simulink model "ARO40506DOF_2020a_2025"  (R2025b)
settings: Solver=FixedStepAuto  StartTime=0.0  StopTime=60  FixedStep=.01  RelTol=1e-3
libraries: simulink_extras x7
settings Model: PacingRate=1000  Creator=Rainman  LastModifiedBy=cdriggs
settings SolverCC: ZeroCrossControl=EnableAll
settings DebuggingCC: SignalInfNanChecking=warning
settings RTWCC: GPUComputeCapability=3.5

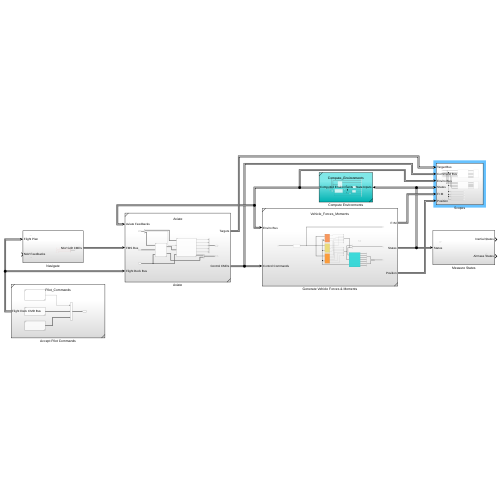
[thumbnail: Simulink's stored preview of the top-level diagram]
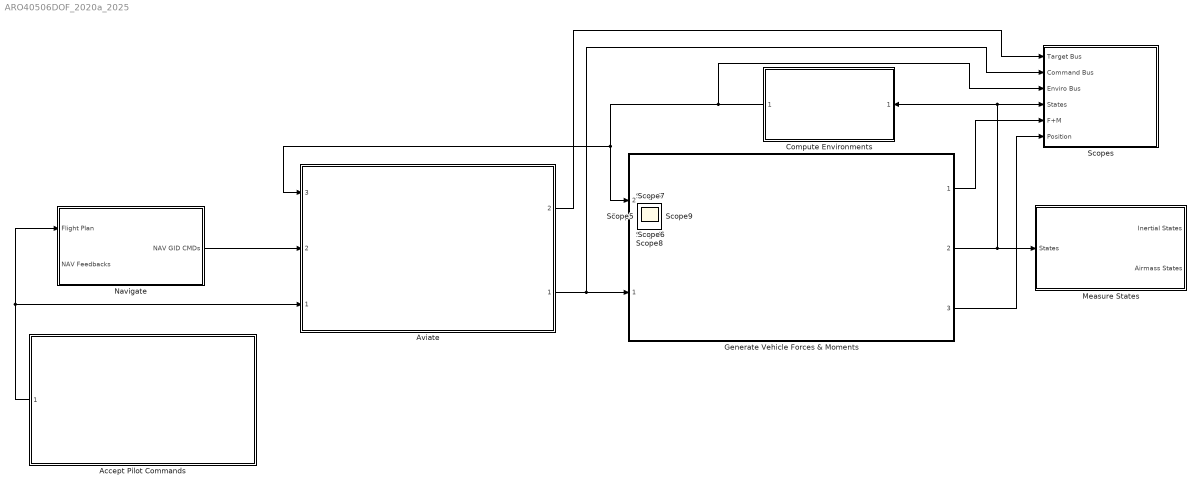
== system ARO40506DOF_2020a_2025 ==
  Accept Pilot Commands : Subsystem  ReferencedSubsystem=Pilot_Commands
  Aviate : Subsystem  ReferencedSubsystem=Aviate
      settings: PortSchema="{\"entries\":[{\"content\":{\"sides\":[{\"content\":{\"connectorIds\":[\"In3\",\"In2\",\"In1\"]},\"type\":\"ConnectorPlacement.EquallySpacedRectSide\",\"uuid\":\"f13bb7a0-c278-4e6a-87bd-80b067821608\"},{\"content\":{\"connectorIds\":[\"Out2\",\"Out1\"],\"side\":\"RIGHT\"},\"type\":\"ConnectorPlacement.EquallySpacedRectSide\",\"uuid\":\"000ddb2c-cb93-4942-87ef-30ae2dcc275e\"},{\"content\":{\"side\":\"TOP\"},\"type\":\"ConnectorPlacement.EquallySpacedRectSide\",\"uuid\":\"c3152a53-2ce1-4a0b-9ad8-bcbeca850b30\"}]},\"type\":\"ConnectorPlacement.EquallySpacedConnector\",\"uuid\":\"e0cd03c4-ca4d-4b0c-94c1-0c67997df9b9\"}],\"packageUris\":[\"http://schema.mathworks.com/mf0/Connector/R2020b\"],\"version\":\"1.0\"}"
  Compute Environments : Subsystem  ReferencedSubsystem=Compute_Environments
  Generate Vehicle Forces & Moments : Subsystem  ReferencedSubsystem=Vehicle_Forces_Moments
      settings: PortSchema="{\"entries\":[{\"content\":{\"sides\":[{\"content\":{\"connectorIds\":[\"In2\",\"In1\"]},\"type\":\"ConnectorPlacement.EquallySpacedRectSide\",\"uuid\":\"c7a215e5-d416-4ad4-83d0-8365272d1a03\"},{\"content\":{\"connectorIds\":[\"Out1\",\"Out2\",\"Out3\"],\"side\":\"RIGHT\"},\"type\":\"ConnectorPlacement.EquallySpacedRectSide\",\"uuid\":\"c94239bd-91e1-4e40-88df-9a8012874706\"},{\"content\":{\"side\":\"TOP\"},\"type\":\"ConnectorPlacement.EquallySpacedRectSide\",\"uuid\":\"517c4bf5-dd91-4ac4-b774-658dcc3846ed\"}]},\"type\":\"ConnectorPlacement.EquallySpacedConnector\",\"uuid\":\"ee7d0a5a-600e-4f04-ae5a-149fcc3f5966\"}],\"packageUris\":[\"http://schema.mathworks.com/mf0/Connector/R2020b\"],\"version\":\"1.0\"}"
  Measure States : Subsystem
  Navigate : Subsystem
  Scopes : Subsystem
  Scope{,1..9} (10 alike) : Scope
      Scope settings: ActiveDisplayYMinimum=824.79015242294952  ActiveDisplayYMaximum=887.11668658276335  DataLoggingVariableName=ScopeData16
      Scope1 settings: ActiveDisplayYMinimum=-0.0918699619645163  ActiveDisplayYMaximum=0.1361905923482078  DataLoggingVariableName=ScopeData17
      Scope2 settings: ActiveDisplayYMinimum=-0.0012525958255160388  ActiveDisplayYMaximum=0.0018610833356130711  DataLoggingVariableName=ScopeData18
      Scope3 settings: ActiveDisplayYMinimum=-1  ActiveDisplayYMaximum=1  DataLoggingVariableName=ScopeData8
      Scope4 settings: ActiveDisplayYMinimum=-1  ActiveDisplayYMaximum=1  DataLoggingVariableName=ScopeData19
      Scope5 settings: ActiveDisplayYMinimum=-1  ActiveDisplayYMaximum=1  DataLoggingVariableName=ScopeData8
      Scope6 settings: ActiveDisplayYMinimum=-1  ActiveDisplayYMaximum=1  DataLoggingVariableName=ScopeData19
      Scope7 settings: ActiveDisplayYMinimum=-10.79844220865172  ActiveDisplayYMaximum=12.310938023183525  DataLoggingVariableName=ScopeData24
      Scope8 settings: ActiveDisplayYMinimum=-2.0057474745908946E-6  ActiveDisplayYMaximum=1.8051727271318056E-5  DataLoggingVariableName=ScopeData25
      Scope9 settings: ActiveDisplayYMinimum=-1.1579459752656034  ActiveDisplayYMaximum=0.3943110608301495  DataLoggingVariableName=ScopeData29
  wires:
  Navigate/1(NAV GID CMDs) -> Aviate/2
  Aviate/1 -> Scopes/2(Command Bus), Generate Vehicle Forces & Moments/1
  Accept Pilot Commands/1 -> Navigate/1(Flight Plan), Aviate/1
  Generate Vehicle Forces & Moments/2 -> Compute Environments/1, Scopes/4(States), Measure States/1(States)
  Compute Environments/1 -> Scopes/3(Enviro Bus), Generate Vehicle Forces & Moments/2, Aviate/3
  Generate Vehicle Forces & Moments/1 -> Scopes/5(F+M)
  Generate Vehicle Forces & Moments/3 -> Scopes/6(Position)
  Aviate/2 -> Scopes/1(Target Bus)

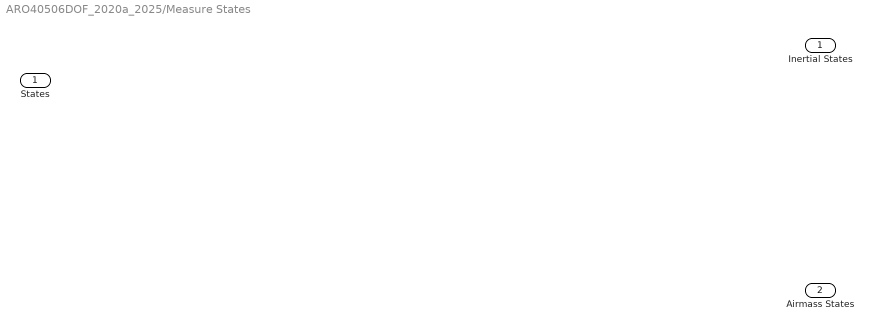
== system ARO40506DOF_2020a_2025/Measure States ==
  States : Inport
  Inertial States : Outport
  Airmass States : Outport  Port=2

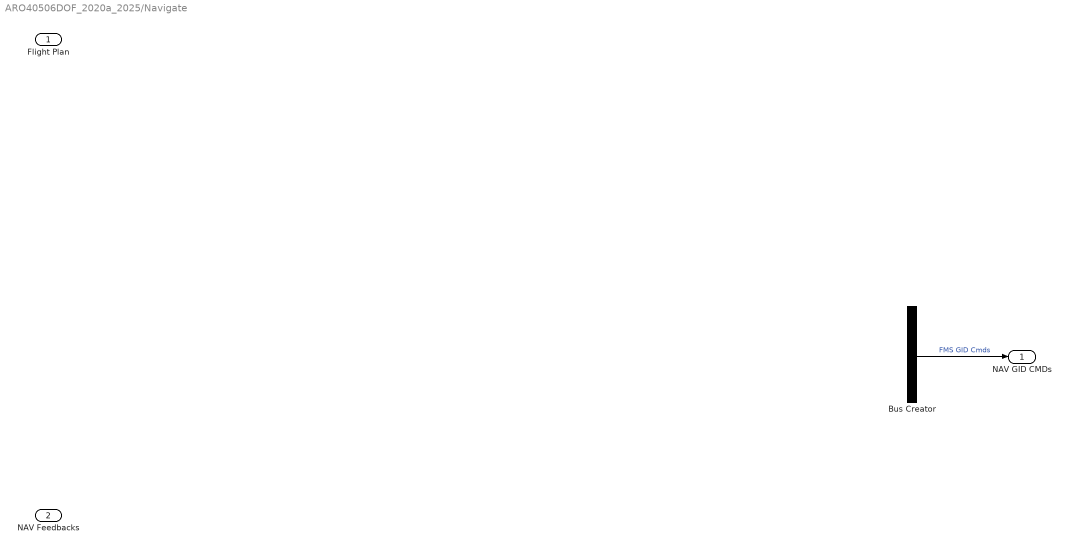
== system ARO40506DOF_2020a_2025/Navigate ==
  Flight Plan : Inport
  NAV Feedbacks : Inport  Port=2
  Bus Creator : BusCreator  Inputs=4
  NAV GID CMDs : Outport
  wires:
  Bus Creator/1 -> NAV GID CMDs/1  "FMS GID Cmds"
  ? -> Bus Creator/1  "FMS ALT Target"
  ? -> Bus Creator/2  "FMS VS Target"
  ? -> Bus Creator/3  "FMS HDG Target"
  ? -> Bus Creator/4  "FMS SPD Target"

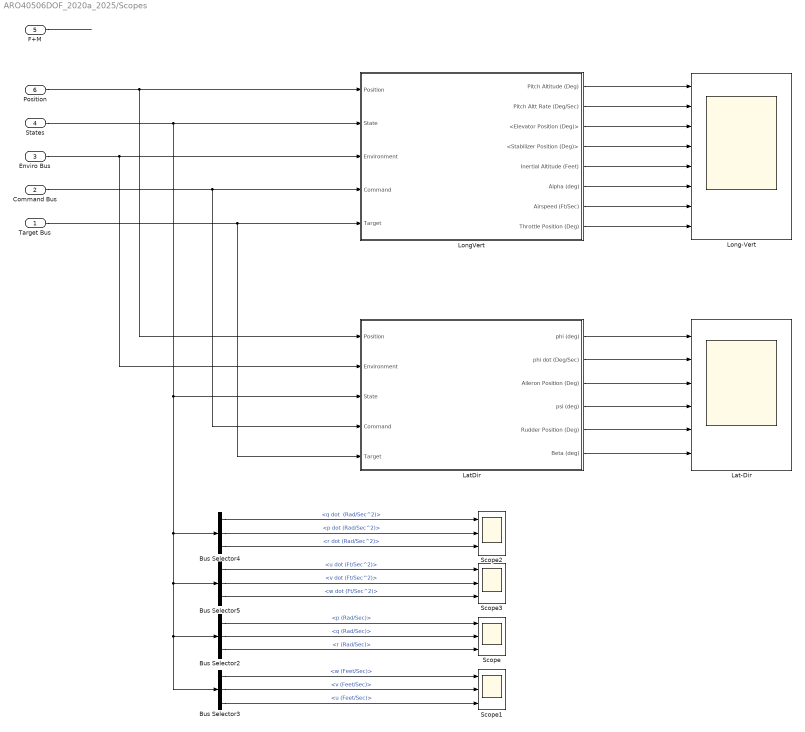
== system ARO40506DOF_2020a_2025/Scopes ==
  Target Bus : Inport
  Command Bus : Inport  Port=2
  Enviro Bus : Inport  Port=3
  States : Inport  Port=4
  F+M : Inport  Port=5
  Position : Inport  Port=6
  Bus Selector2 : BusSelector  OutputSignals=Rotat.Body.Rates (Rad/Sec).p (Rad/Sec),Rotat.Body.Rates (Rad/Sec).q (Rad/Sec),Rotat.Body.Rates (Rad/Sec).r (Rad/Sec)
  Bus Selector3 : BusSelector  OutputSignals=Trans.Body Veloc.w (Feet/Sec),Trans.Body Veloc.v (Feet/Sec),Trans.Body Veloc.u (Feet/Sec)
  Bus Selector4 : BusSelector  OutputSignals="Rotat.Body.Accelerations (Rad/Sec^2).q dot  (Rad/Sec^2),Rotat.Body.Accelerations (Rad/Sec^2).p dot (Rad/Sec^2),Rotat.Body.Accelerations (Rad/Sec^2).r dot (Rad/Sec^2)"
  Bus Selector5 : BusSelector  OutputSignals=Trans.Lin Accels.u dot (Ft/Sec^2),Trans.Lin Accels.v dot (Ft/Sec^2),Trans.Lin Accels.w dot (Ft/Sec^2)
  Lat-Dir : Scope  NumInputPorts=6
      settings: ActiveDisplayYMinimum=-6.499523495214234  ActiveDisplayYMaximum=17.811539807152641
  LatDir : Subsystem
  Long-Vert : Scope  NumInputPorts=8
      settings: ActiveDisplayYMinimum=-0.011330669657011287  ActiveDisplayYMaximum=0.010438336756237168
  LongVert : Subsystem
  Scope{,1..3} (4 alike) : Scope  NumInputPorts=3
      Scope settings: ActiveDisplayYMinimum=-5.25071638692835E-14  ActiveDisplayYMaximum=8.1502400193216538E-14  DataLoggingVariableName=ScopeData2
      Scope1 settings: ActiveDisplayYMinimum=-80.784705727324493  ActiveDisplayYMaximum=49.537985206955256  DataLoggingVariableName=ScopeData3
      Scope2 settings: ActiveDisplayYMinimum=-0.010938926120745193  ActiveDisplayYMaximum=0.089546281056735608  DataLoggingVariableName=ScopeData6
      Scope3 settings: ActiveDisplayYMinimum=-7.3926575931100222  ActiveDisplayYMaximum=3.2145324083165696  DataLoggingVariableName=ScopeData9
  wires:
  States/1 -> LongVert/2(State), LatDir/3(State), Bus Selector4/1, Bus Selector5/1, Bus Selector2/1, Bus Selector3/1
  Enviro Bus/1 -> LatDir/2(Environment), LongVert/3(Environment)
  Bus Selector2/1 -> Scope/1  "<p (Rad/Sec)>"
  Bus Selector2/2 -> Scope/2  "<q (Rad/Sec)>"
  Bus Selector2/3 -> Scope/3  "<r (Rad/Sec)>"
  Bus Selector3/1 -> Scope1/1  "<w (Feet/Sec)>"
  Bus Selector3/2 -> Scope1/2  "<v (Feet/Sec)>"
  Bus Selector3/3 -> Scope1/3  "<u (Feet/Sec)>"
  Bus Selector4/2 -> Scope2/2  "<p dot (Rad/Sec^2)>"
  Bus Selector4/3 -> Scope2/3  "<r dot (Rad/Sec^2)>"
  Bus Selector4/1 -> Scope2/1  "<q dot  (Rad/Sec^2)>"
  Bus Selector5/1 -> Scope3/1  "<u dot (Ft/Sec^2)>"
  Bus Selector5/2 -> Scope3/2  "<v dot (Ft/Sec^2)>"
  Bus Selector5/3 -> Scope3/3  "<w dot (Ft/Sec^2)>"
  F+M/1 -> ?
  Position/1 -> LatDir/1(Position), LongVert/1(Position)
  LongVert/1(Pitch Altitude (Deg)) -> Long-Vert/1
  LongVert/2(Pitch Altt Rate (Deg/Sec)) -> Long-Vert/2
  LongVert/3(<Elevator Position (Deg)>) -> Long-Vert/3
  LongVert/4(<Stabilizer Position (Deg)>) -> Long-Vert/4
  LongVert/5(Inertial Altitude (Feet)) -> Long-Vert/5
  LongVert/6(Alpha (deg)) -> Long-Vert/6
  LongVert/7(Airspeed (Ft/Sec)) -> Long-Vert/7
  LongVert/8(Throttle Position (Deg)) -> Long-Vert/8
  LatDir/1(phi (deg)) -> Lat-Dir/1
  LatDir/2(phi dot (Deg/Sec)) -> Lat-Dir/2
  LatDir/3(Aileron Position (Deg)) -> Lat-Dir/3
  LatDir/4(psi (deg)) -> Lat-Dir/4
  LatDir/5(Rudder Position (Deg)) -> Lat-Dir/5
  LatDir/6(Beta (deg)) -> Lat-Dir/6
  Command Bus/1 -> LongVert/4(Command), LatDir/4(Command)
  Target Bus/1 -> LatDir/5(Target), LongVert/5("Target ")

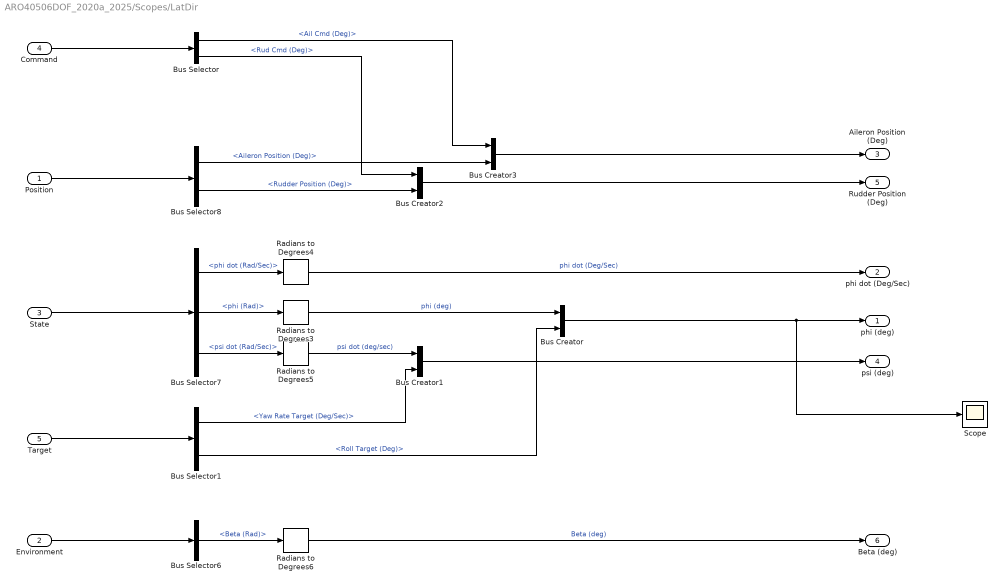
== system ARO40506DOF_2020a_2025/Scopes/LatDir ==
  Position : Inport
  Environment : Inport  Port=2
  State : Inport  Port=3
  Command : Inport  Port=4
  Target : Inport  Port=5
  Bus Creator{,1..3} (4 alike) : BusCreator  Inputs=2
  Bus Selector : BusSelector  OutputSignals=Ail Cmd (Deg),Rud Cmd (Deg)
  Bus Selector1 : BusSelector  OutputSignals=signal1.Yaw Rate Target (Deg/Sec),signal1.Roll Target (Deg)
  Bus Selector6 : BusSelector  OutputSignals=Aero angles.Beta (Rad)
  Bus Selector7 : BusSelector  OutputSignals=Rotat.Attitude Rates.phi dot (Rad/Sec),Rotat.Attitude.phi (Rad),Rotat.Attitude Rates.psi dot (Rad/Sec)
  Bus Selector8 : BusSelector  OutputSignals=Aileron Position (Deg),Rudder Position (Deg)
  Radians to Degrees{3..6} (4 alike) : simulink_extras/Transformations/Radians to Degrees
  Scope : Scope
      settings: ActiveDisplayYMinimum=-1  ActiveDisplayYMaximum=1  DataLoggingVariableName=ScopeData27
  phi (deg) : Outport
  phi dot (Deg/Sec) : Outport  Port=2
  Aileron Position (Deg) : Outport  Port=3
  psi (deg) : Outport  Port=4
  Rudder Position (Deg) : Outport  Port=5
  Beta (deg) : Outport  Port=6
  wires:
  Radians to Degrees3/1 -> Bus Creator/1  "phi (deg)"
  Bus Creator1/1 -> psi (deg)/1
  Bus Selector/1 -> Bus Creator3/1  "<Ail Cmd (Deg)>"
  Bus Selector6/1 -> Radians to Degrees6/1  "<Beta (Rad)>"
  Bus Selector7/2 -> Radians to Degrees3/1  "<phi (Rad)>"
  Radians to Degrees5/1 -> Bus Creator1/1  "psi dot (deg/sec)"
  Bus Selector8/2 -> Bus Creator2/2  "<Rudder Position (Deg)>"
  Bus Selector7/3 -> Radians to Degrees5/1  "<psi dot (Rad/Sec)>"
  Bus Selector7/1 -> Radians to Degrees4/1  "<phi dot (Rad/Sec)>"
  Bus Selector8/1 -> Bus Creator3/2  "<Aileron Position (Deg)>"
  Bus Creator2/1 -> Rudder Position (Deg)/1
  Radians to Degrees6/1 -> Beta (deg)/1  "Beta (deg)"
  Radians to Degrees4/1 -> phi dot (Deg/Sec)/1  "phi dot (Deg/Sec)"
  Bus Creator/1 -> Scope/1, phi (deg)/1
  State/1 -> Bus Selector7/1
  Bus Creator3/1 -> Aileron Position (Deg)/1
  Bus Selector1/1 -> Bus Creator1/2  "<Yaw Rate Target (Deg/Sec)>"
  Environment/1 -> Bus Selector6/1
  Position/1 -> Bus Selector8/1
  Target/1 -> Bus Selector1/1
  Command/1 -> Bus Selector/1
  Bus Selector/2 -> Bus Creator2/1  "<Rud Cmd (Deg)>"
  Bus Selector1/2 -> Bus Creator/2  "<Roll Target (Deg)>"

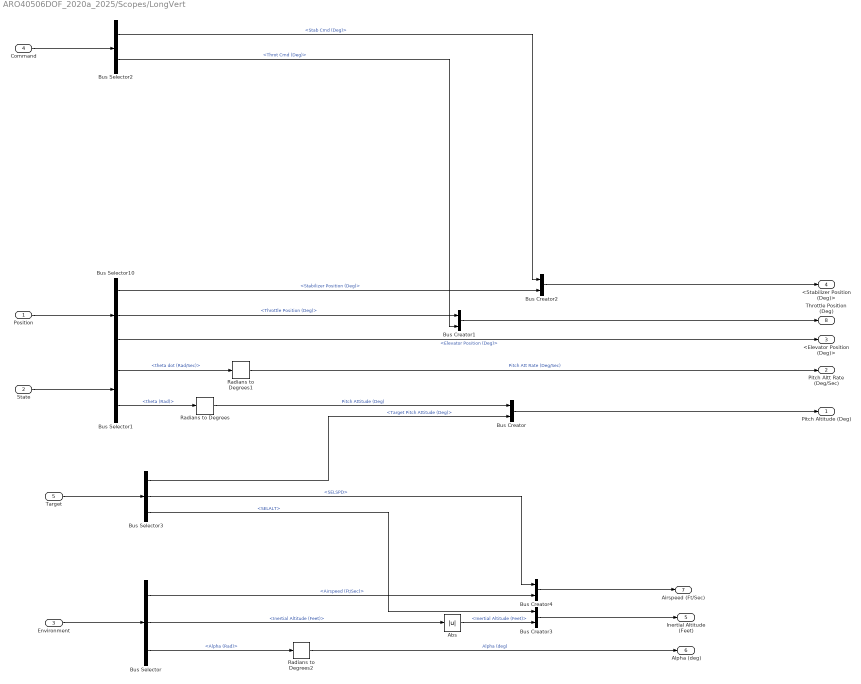
== system ARO40506DOF_2020a_2025/Scopes/LongVert ==
  Position : Inport
  State : Inport  Port=2
  Environment : Inport  Port=3
  Command : Inport  Port=4
  "Target " : Inport  Port=5
  Abs : Abs  SaturateOnIntegerOverflow=off
  Bus Creator{,1..4} (5 alike) : BusCreator  Inputs=2
  Bus Selector : BusSelector  OutputSignals=Airspeed (Ft/Sec),Trans.Inertial Pos.Inertial Altitude (Feet),Aero angles.Alpha (Rad)
  Bus Selector1 : BusSelector  OutputSignals=Rotat.Attitude Rates.theta dot (Rad/Sec),Rotat.Attitude.theta (Rad)
  Bus Selector10 : BusSelector  OutputSignals=Stabilizer Position (Deg),Throttle Position (Deg),Elevator Position (Deg)
  Bus Selector2 : BusSelector  OutputSignals=Stab Cmd (Deg),Throt Cmd (Deg)
  Bus Selector3 : BusSelector  OutputSignals=signal1.Target Pitch Attitude (Deg),signal2.SELSPD,signal2.SELALT
  Radians to Degrees : simulink_extras/Transformations/Radians to Degrees
  Radians to Degrees1 : simulink_extras/Transformations/Radians to Degrees
  Radians to Degrees2 : simulink_extras/Transformations/Radians to Degrees
  Pitch Altitude (Deg) : Outport
  Pitch Altt Rate (Deg/Sec) : Outport  Port=2
  <Elevator Position (Deg)> : Outport  Port=3
  <Stabilizer Position (Deg)> : Outport  Port=4
  Inertial Altitude (Feet) : Outport  Port=5
  Alpha (deg) : Outport  Port=6
  Airspeed (Ft/Sec) : Outport  Port=7
  Throttle Position (Deg) : Outport  Port=8
  wires:
  Radians to Degrees/1 -> Bus Creator/1  "Pitch Attitude (Deg)"
  Bus Selector/3 -> Radians to Degrees2/1  "<Alpha (Rad)>"
  Bus Selector1/2 -> Radians to Degrees/1  "<theta (Rad)>"
  Abs/1 -> Bus Creator3/2  "<Inertial Altitude (Feet)>"
  Radians to Degrees1/1 -> Pitch Altt Rate (Deg/Sec)/1  "Pitch Att Rate (Deg/Sec)"
  Bus Selector/1 -> Bus Creator4/2  "<Airspeed (Ft/Sec)>"
  Bus Selector1/1 -> Radians to Degrees1/1  "<theta dot (Rad/Sec)>"
  Bus Selector/2 -> Abs/1  "<Inertial Altitude (Feet)>"
  Bus Selector3/3 -> Bus Creator3/1  "<SELALT>"
  Bus Selector10/2 -> Bus Creator1/1  "<Throttle Position (Deg)>"
  Environment/1 -> Bus Selector/1
  Bus Creator2/1 -> <Stabilizer Position (Deg)>/1
  Position/1 -> Bus Selector10/1
  Bus Creator3/1 -> Inertial Altitude (Feet)/1
  Bus Selector10/1 -> Bus Creator2/2  "<Stabilizer Position (Deg)>"
  Radians to Degrees2/1 -> Alpha (deg)/1  "Alpha (deg)"
  Bus Selector3/1 -> Bus Creator/2  "<Target Pitch Attitude (Deg)>"
  Bus Creator1/1 -> Throttle Position (Deg)/1
  Bus Creator/1 -> Pitch Altitude (Deg)/1
  Bus Selector10/3 -> <Elevator Position (Deg)>/1  "<Elevator Position (Deg)>"
  Bus Selector3/2 -> Bus Creator4/1  "<SELSPD>"
  State/1 -> Bus Selector1/1
  Bus Creator4/1 -> Airspeed (Ft/Sec)/1
  "Target "/1 -> Bus Selector3/1
  Command/1 -> Bus Selector2/1
  Bus Selector2/1 -> Bus Creator2/1  "<Stab Cmd (Deg)>"
  Bus Selector2/2 -> Bus Creator1/2  "<Throt Cmd (Deg)>"
